simulink model "FeedbackSim"  (R2018b)
settings: Solver=VariableStepAuto  StartTime=0.0  StopTime=10.0  RelTol=1e-3
values from neighbouring files (symbols this model uses):
  g = 9.81    [BasePendulumTest.m]    (also in FeedbackSimOptimization.m; FeedbackSimTest.m; SimVariables.mat)
  ICs = [pi 0]    [BasePendulumTest.m]    (also in FeedbackSimOptimization.m; FeedbackSimTest.m; SimVariables.mat = [3.14159265359 0])
  ka = 1    [FeedbackSimOptimization.m]    (also in RunFBSim_Opt.m = x(1))
  kp = 1    [FeedbackSimOptimization.m]    (also in RunFBSim_Opt.m = x(3))
  kv = 1    [FeedbackSimOptimization.m]    (also in RunFBSim_Opt.m = x(2))
  L = 0.2    [BasePendulumTest.m]    (also in FeedbackSimOptimization.m; FeedbackSimTest.m; SimVariables.mat)
  lambda = 31/1000    (= 0.031)    [FeedbackSimOptimization.m]    (also in SimVariables.mat)
  m = 4    [BasePendulumTest.m]    (also in FeedbackSimOptimization.m; FeedbackSimTest.m; SimVariables.mat)
  PertAmplitude = -1*[0 1 2 5]    [BasePendulumTest.m]    (also in FeedbackSimOptimization.m = -0.1; FeedbackSimTest.m = 0; SimVariables.mat = -0.1)
  PertDelay_Acc = 0.1    [FeedbackSimOptimization.m]    (also in SimVariables.mat)
  PertDelay_DeAcc = 0.6    [FeedbackSimOptimization.m]    (also in SimVariables.mat)
  PertPeriod = time(end)    [BasePendulumTest.m]    (also in FeedbackSimOptimization.m; FeedbackSimTest.m; SimVariables.mat = 1)
  PertWidth = 5    [BasePendulumTest.m]    (also in FeedbackSimOptimization.m = 10; FeedbackSimTest.m = 10; SimVariables.mat = 10)
  tau = 40/1000    (= 0.04)    [FeedbackSimOptimization.m]    (also in SimVariables.mat)
settings Model: Creator=seboe  LastModifiedBy=seboe

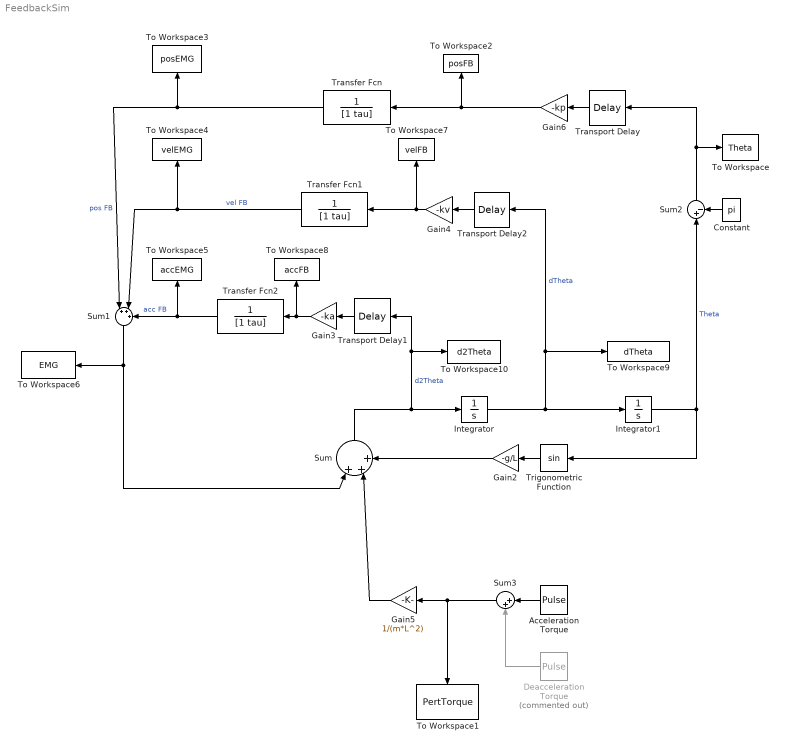
== system FeedbackSim ==
  Acceleration Torque : DiscretePulseGenerator  PulseType=Time based  Amplitude=PertAmplitude  Period=PertPeriod  PulseWidth=PertWidth  PhaseDelay=PertDelay_Acc
  Constant : Constant  Value=pi
  Deacceleration Torque : DiscretePulseGenerator  Commented=on  PulseType=Time based  Amplitude=-PertAmplitude  Period=PertPeriod  PulseWidth=PertWidth  PhaseDelay=PertDelay_DeAcc
  Gain2 : Gain  Gain=-g/L
  Gain3 : Gain  Gain=-ka
  Gain4 : Gain  Gain=-kv
  Gain5 : Gain  Gain=1/(m*L^2)
  Gain6 : Gain  Gain=-kp
  Integrator : Integrator  InitialCondition=ICs(2)
  Integrator1 : Integrator  InitialCondition=ICs(1)
  Sum : Sum  Inputs=|+++
  Sum1 : Sum  Inputs=|+++
  Sum2 : Sum  Inputs=|+-
  Sum3 : Sum  Inputs=|++
  To Workspace : ToWorkspace  VariableName=Theta  SaveFormat=Timeseries  SampleTime=-1
  To Workspace1 : ToWorkspace  VariableName=PertTorque  SaveFormat=Timeseries  SampleTime=-1
  To Workspace10 : ToWorkspace  VariableName=d2Theta  SaveFormat=Timeseries  SampleTime=-1
  To Workspace2 : ToWorkspace  VariableName=posFB  SaveFormat=Timeseries  SampleTime=-1
  To Workspace3 : ToWorkspace  VariableName=posEMG  SaveFormat=Timeseries  SampleTime=-1
  To Workspace4 : ToWorkspace  VariableName=velEMG  SaveFormat=Timeseries  SampleTime=-1
  To Workspace5 : ToWorkspace  VariableName=accEMG  SaveFormat=Timeseries  SampleTime=-1
  To Workspace6 : ToWorkspace  VariableName=EMG  SaveFormat=Timeseries  SampleTime=-1
  To Workspace7 : ToWorkspace  VariableName=velFB  SaveFormat=Timeseries  SampleTime=-1
  To Workspace8 : ToWorkspace  VariableName=accFB  SaveFormat=Timeseries  SampleTime=-1
  To Workspace9 : ToWorkspace  VariableName=dTheta  SaveFormat=Timeseries  SampleTime=-1
  Transfer Fcn : TransferFcn  Denominator=[1 tau]
  Transfer Fcn1 : TransferFcn  Denominator=[1 tau]
  Transfer Fcn2 : TransferFcn  Denominator=[1 tau]
  Transport Delay : TransportDelay  DelayTime=lambda
  Transport Delay1 : TransportDelay  DelayTime=lambda
  Transport Delay2 : TransportDelay  DelayTime=lambda
  Trigonometric Function : Trigonometry
  wires:
  Sum/1 -> Integrator/1, Transport Delay1/1, To Workspace10/1  "d2Theta"
  Trigonometric Function/1 -> Gain2/1
  Gain5/1 -> Sum/2
  Gain2/1 -> Sum/3
  Acceleration Torque/1 -> Sum3/1
  Integrator1/1 -> Sum2/1, Trigonometric Function/1  "Theta"
  Integrator/1 -> Transport Delay2/1, To Workspace9/1, Integrator1/1  "dTheta"
  Transport Delay/1 -> Gain6/1
  Transport Delay2/1 -> Gain4/1
  Transport Delay1/1 -> Gain3/1
  Sum1/1 -> Sum/1, To Workspace6/1
  Gain3/1 -> To Workspace8/1, Transfer Fcn2/1
  Gain4/1 -> To Workspace7/1, Transfer Fcn1/1
  Gain6/1 -> Transfer Fcn/1, To Workspace2/1
  Transfer Fcn2/1 -> Sum1/3, To Workspace5/1  "acc FB"
  Transfer Fcn1/1 -> To Workspace4/1, Sum1/2  "vel FB"
  Transfer Fcn/1 -> Sum1/1, To Workspace3/1  "pos FB"
  Constant/1 -> Sum2/2
  Sum2/1 -> To Workspace/1, Transport Delay/1
  Sum3/1 -> To Workspace1/1, Gain5/1
  Deacceleration Torque/1 -> Sum3/2
